simulink model "FPU_sim_out"  (Simulink 7.6)
settings: Solver=FixedStepDiscrete  StartTime=0.0  StopTime=200  FixedStep=1  RelTol=1e-3
libraries: simulink x24
settings Model: Creator=jordan  LastModifiedBy=jordan
settings OptimizationCC: BlockReduction=off  ConditionallyExecuteInputs=off

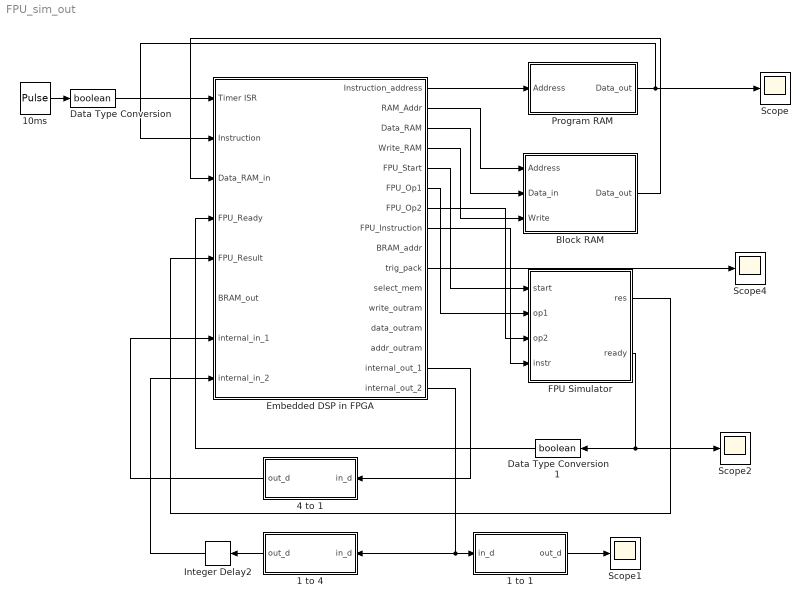
== system FPU_sim_out ==
  1 to 1 : Stateflow chart  TreatAsAtomicUnit=on
  1 to 4 : Stateflow chart  TreatAsAtomicUnit=on
  10ms : DiscretePulseGenerator  Period=50
  4 to 1 : Stateflow chart  TreatAsAtomicUnit=on
  Block RAM : Subsystem
  Data Type Conversion : DataTypeConversion  OutDataTypeStr=boolean
  Data Type Conversion1 : DataTypeConversion  OutDataTypeStr=boolean
  Embedded DSP in FPGA : Subsystem
  FPU Simulator : Stateflow chart  TreatAsAtomicUnit=on
  Integer Delay2 : simulink/Discrete/Integer Delay  NumDelays=1  vinit=0.0  samptime=-1
  Program RAM : Subsystem
  Scope{,1..2,4} (4 alike) : Scope
      Scope settings: MaxDataPoints=50000
      Scope1 settings: SaveName=ScopeData5  MaxDataPoints=50000
      Scope2 settings: SaveName=ScopeData4  MaxDataPoints=50000
      Scope4 settings: SaveName=ScopeData13  MaxDataPoints=50000
  wires:
  10ms/1 -> Data Type Conversion/1
  Data Type Conversion/1 -> Embedded DSP in FPGA/1(Timer ISR)
  Embedded DSP in FPGA/1(Instruction_address) -> Program RAM/1(Address)
  Program RAM/1(Data_out) -> Embedded DSP in FPGA/2(Instruction), Scope/1
  Embedded DSP in FPGA/2(RAM_Addr) -> Block RAM/1(Address)
  Embedded DSP in FPGA/3(Data_RAM) -> Block RAM/2(Data_in)
  Embedded DSP in FPGA/4(Write_RAM) -> Block RAM/3(Write)
  Block RAM/1(Data_out) -> Embedded DSP in FPGA/3(Data_RAM_in)
  Embedded DSP in FPGA/5(FPU_Start) -> FPU Simulator/1(start)
  Embedded DSP in FPGA/6(FPU_Op1) -> FPU Simulator/2(op1)
  Embedded DSP in FPGA/7(FPU_Op2) -> FPU Simulator/3(op2)
  Embedded DSP in FPGA/8(FPU_Instruction) -> FPU Simulator/4(instr)
  FPU Simulator/2(ready) -> Scope2/1, Data Type Conversion1/1
  FPU Simulator/1(res) -> Embedded DSP in FPGA/5(FPU_Result)
  Data Type Conversion1/1 -> Embedded DSP in FPGA/4(FPU_Ready)
  Embedded DSP in FPGA/15(internal_out_1) -> 4 to 1/1(in_d)
  4 to 1/1(out_d) -> Embedded DSP in FPGA/7(internal_in_1)
  Embedded DSP in FPGA/16(internal_out_2) -> 1 to 4/1(in_d), 1 to 1/1(in_d)
  1 to 4/1(out_d) -> Integer Delay2/1
  Integer Delay2/1 -> Embedded DSP in FPGA/8(internal_in_2)
  1 to 1/1(out_d) -> Scope1/1
  Embedded DSP in FPGA/10(trig_pack) -> Scope4/1

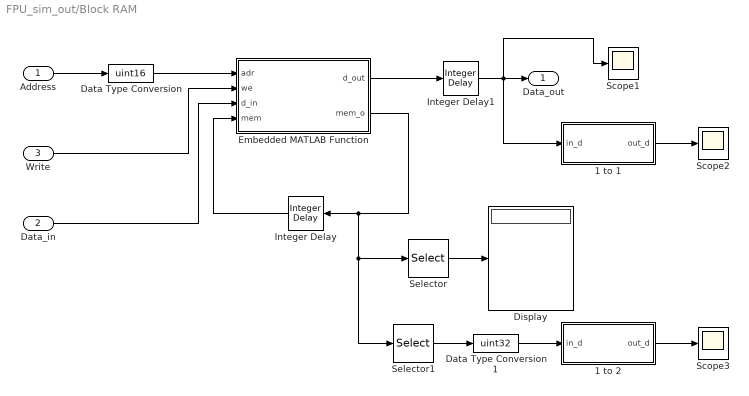
== system FPU_sim_out/Block RAM ==
  Address : Inport  OutDataTypeStr=fixdt(0,12,0)
  Data_in : Inport  Port=2  OutDataTypeStr=uint32
  Write : Inport  Port=3  OutDataTypeStr=boolean
  1 to 1 : Stateflow chart  TreatAsAtomicUnit=on
  1 to 2 : Stateflow chart  TreatAsAtomicUnit=on
  Data Type Conversion : DataTypeConversion  OutDataTypeStr=uint16
  Data Type Conversion1 : DataTypeConversion  OutDataTypeStr=uint32
  Display : Display
  Embedded MATLAB Function : Stateflow chart  TreatAsAtomicUnit=on
  Integer Delay : simulink/Discrete/Integer Delay  NumDelays=1  vinit=zeros(1,100)  samptime=-1
  Integer Delay1 : simulink/Discrete/Integer Delay  NumDelays=1  vinit=0.0  samptime=-1
  Scope1 : Scope
      settings: SaveName=ScopeData23  MaxDataPoints=50000
  Scope2 : Scope
      settings: SaveName=ScopeData14  MaxDataPoints=50000
  Scope3 : Scope
      settings: SaveName=ScopeData31  MaxDataPoints=50000
  Selector : Selector  InputPortWidth=100  IndexOptions=Index vector (dialog)  Indices=1:5  OutputSizes=1
  Selector1 : Selector  InputPortWidth=100  IndexOptions=Index vector (dialog)  Indices=5  OutputSizes=1
  Data_out : Outport  OutDataTypeStr=uint32
  wires:
  Address/1 -> Data Type Conversion/1
  Write/1 -> Embedded MATLAB Function/2(we)
  Data_in/1 -> Embedded MATLAB Function/3(d_in)
  Embedded MATLAB Function/1(d_out) -> Integer Delay1/1
  Integer Delay/1 -> Embedded MATLAB Function/4(mem)
  Embedded MATLAB Function/2(mem_o) -> Integer Delay/1, Selector/1, Selector1/1
  Data Type Conversion/1 -> Embedded MATLAB Function/1(adr)
  Integer Delay1/1 -> Data_out/1, Scope1/1, 1 to 1/1(in_d)
  Selector/1 -> Display/1
  1 to 1/1(out_d) -> Scope2/1
  1 to 2/1(out_d) -> Scope3/1
  Selector1/1 -> Data Type Conversion1/1
  Data Type Conversion1/1 -> 1 to 2/1(in_d)

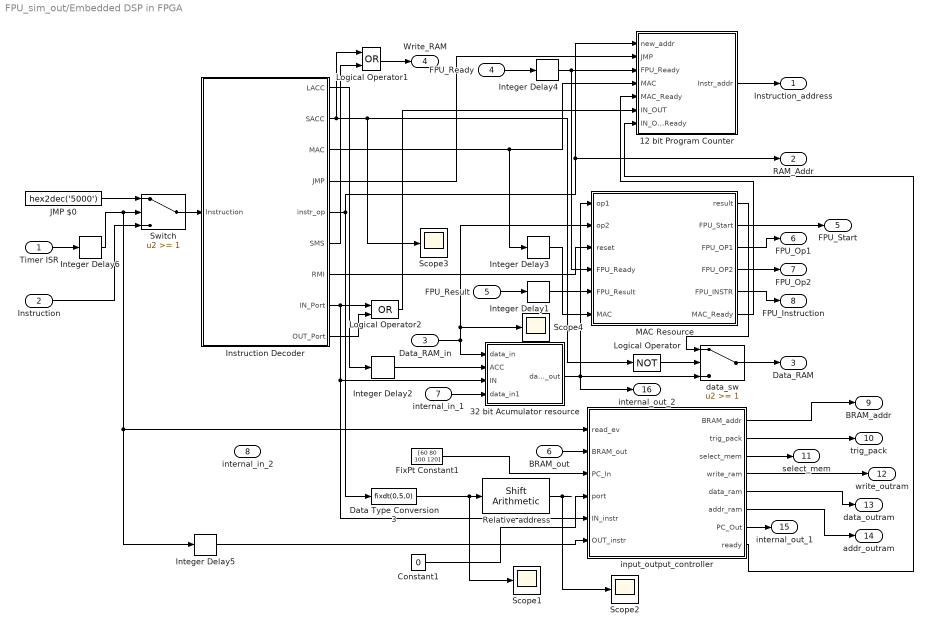
== system FPU_sim_out/Embedded DSP in FPGA ==
  Timer ISR : Inport  OutDataTypeStr=boolean
  Instruction : Inport  Port=2  OutDataTypeStr=uint16
  Data_RAM_in : Inport  Port=3  OutDataTypeStr=uint32
  FPU_Ready : Inport  Port=4  OutDataTypeStr=boolean
  FPU_Result : Inport  Port=5  OutDataTypeStr=uint32
  BRAM_out : Inport  Port=6  OutDataTypeStr=uint8
  internal_in_1 : Inport  Port=7  OutDataTypeStr=uint32
  internal_in_2 : Inport  Port=8
  12 bit Program Counter : Subsystem
  32 bit Acumulator resource : Subsystem
  Constant1 : Constant  Value=0  OutDataTypeStr=fixdt(0,5,0)
  Data Type Conversion3 : DataTypeConversion  OutDataTypeStr=fixdt(0,5,0)
  FixPt Constant1 : Constant  DisableCoverage=on  Value=[60 80 100 120]  OutDataTypeStr=uint8
  Instruction Decoder : Subsystem
  Integer Delay{1..4,6} (5 alike) : simulink/Discrete/Integer Delay  NumDelays=1  vinit=0.0  samptime=-1
  Integer Delay5 : simulink/Discrete/Integer Delay  NumDelays=4  vinit=0.0  samptime=-1
  JMP $0 : Constant  DisableCoverage=on  Value=hex2dec('5000')  OutDataTypeStr=Inherit: Inherit via back propagation
  Logical Operator : Logic  Operator=NOT  AllPortsSameDT=off  OutDataTypeStr=boolean
  Logical Operator1 : Logic  Operator=OR  AllPortsSameDT=off  OutDataTypeStr=boolean
  Logical Operator2 : Logic  Operator=OR  AllPortsSameDT=off  OutDataTypeStr=boolean
  MAC Resource : Stateflow chart  TreatAsAtomicUnit=on
  Relative address : simulink/Logic and Bit Operations/Shift Arithmetic  SystemSampleTime=-1  nBitShiftRight=-2  nBinPtShiftRight=0
  Scope{1..4} (4 alike) : Scope
      Scope1 settings: SaveName=ScopeData18  MaxDataPoints=50000
      Scope2 settings: SaveName=ScopeData17  MaxDataPoints=50000
      Scope3 settings: SaveName=ScopeData25  MaxDataPoints=50000
      Scope4 settings: SaveName=ScopeData24  MaxDataPoints=50000
  Switch : Switch  Threshold=1
  data_sw : Switch  Threshold=1
  input_output_controller : Stateflow chart  TreatAsAtomicUnit=on
  Instruction_address : Outport  OutDataTypeStr=fixdt(0,12,0)
  RAM_Addr : Outport  Port=2  OutDataTypeStr=fixdt(0,12,0)
  Data_RAM : Outport  Port=3  OutDataTypeStr=uint32
  Write_RAM : Outport  Port=4  OutDataTypeStr=boolean
  FPU_Start : Outport  Port=5  OutDataTypeStr=boolean
  FPU_Op1 : Outport  Port=6  OutDataTypeStr=uint32
  FPU_Op2 : Outport  Port=7  OutDataTypeStr=uint32
  FPU_Instruction : Outport  Port=8  OutDataTypeStr=fixdt(0,3,0)
  BRAM_addr : Outport  Port=9
  trig_pack : Outport  Port=10
  select_mem : Outport  Port=11
  write_outram : Outport  Port=12
  data_outram : Outport  Port=13
  addr_outram : Outport  Port=14
  internal_out_1 : Outport  Port=15
  internal_out_2 : Outport  Port=16  OutDataTypeStr=uint32
  wires:
  MAC Resource/1(result) -> data_sw/1
  32 bit Acumulator resource/1(data_out) -> MAC Resource/1(op1), data_sw/3, internal_out_2/1
  Data_RAM_in/1 -> 32 bit Acumulator resource/1(data_in), MAC Resource/2(op2), Scope4/1
  Instruction Decoder/5(instr_op) -> 12 bit Program Counter/1(new_addr), RAM_Addr/1, Data Type Conversion3/1
  Instruction Decoder/1(LACC) -> Integer Delay2/1
  Integer Delay2/1 -> 32 bit Acumulator resource/2(ACC)
  Instruction Decoder/2(SACC) -> Logical Operator1/1, Logical Operator/1, Scope3/1
  Logical Operator/1 -> data_sw/2
  Instruction Decoder/4(JMP) -> 12 bit Program Counter/2(JMP)
  Instruction Decoder/3(MAC) -> Integer Delay3/1, 12 bit Program Counter/4(MAC)
  Integer Delay3/1 -> MAC Resource/6(MAC)
  Instruction Decoder/7(RMI) -> MAC Resource/3(reset)
  Instruction Decoder/6(SMS) -> Logical Operator1/2
  Instruction Decoder/8(IN_Port) -> input_output_controller/5(IN_instr), 32 bit Acumulator resource/3(IN), Logical Operator2/1
  Data Type Conversion3/1 -> Relative address/1, Scope1/1
  Switch/1 -> Instruction Decoder/1(Instruction)
  JMP $0/1 -> Switch/1
  12 bit Program Counter/1(Instr_addr) -> Instruction_address/1
  Timer ISR/1 -> Integer Delay6/1
  Instruction/1 -> Switch/3
  data_sw/1 -> Data_RAM/1
  Logical Operator1/1 -> Write_RAM/1
  FPU_Ready/1 -> Integer Delay4/1
  FPU_Result/1 -> Integer Delay1/1
  MAC Resource/3(FPU_OP1) -> FPU_Op1/1
  MAC Resource/4(FPU_OP2) -> FPU_Op2/1
  MAC Resource/5(FPU_INSTR) -> FPU_Instruction/1
  MAC Resource/2(FPU_Start) -> FPU_Start/1
  Integer Delay4/1 -> 12 bit Program Counter/3(FPU_Ready), MAC Resource/4(FPU_Ready)
  Instruction Decoder/9(OUT_Port) -> Logical Operator2/2
  BRAM_out/1 -> input_output_controller/2(BRAM_out)
  input_output_controller/6(addr_ram) -> addr_outram/1
  input_output_controller/4(write_ram) -> write_outram/1
  input_output_controller/5(data_ram) -> data_outram/1
  input_output_controller/1(BRAM_addr) -> BRAM_addr/1
  input_output_controller/2(trig_pack) -> trig_pack/1
  input_output_controller/3(select_mem) -> select_mem/1
  Relative address/1 -> Scope2/1
  input_output_controller/8(ready) -> 12 bit Program Counter/7(IN_OUT_Ready)
  MAC Resource/6(MAC_Ready) -> 12 bit Program Counter/5(MAC_Ready)
  Logical Operator2/1 -> 12 bit Program Counter/6(IN_OUT)
  input_output_controller/7(PC_Out) -> internal_out_1/1
  internal_in_1/1 -> 32 bit Acumulator resource/4(data_in1)
  Integer Delay1/1 -> MAC Resource/5(FPU_Result)
  FixPt Constant1/1 -> input_output_controller/3(PC_In)
  Constant1/1 -> input_output_controller/4(port)
  Integer Delay6/1 -> Switch/2, input_output_controller/1(read_ev), Integer Delay5/1
  Integer Delay5/1 -> input_output_controller/6(OUT_instr)

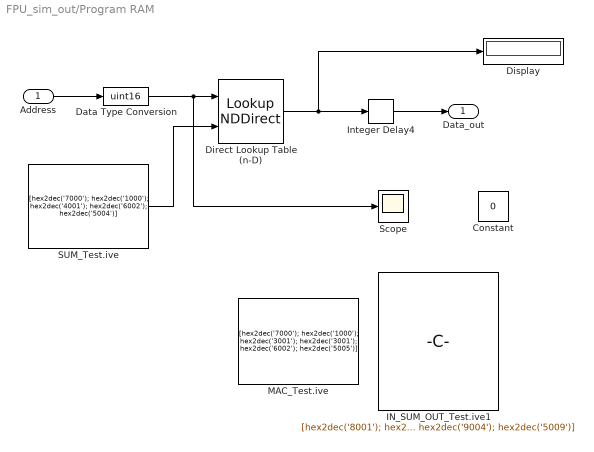
== system FPU_sim_out/Program RAM ==
  Address : Inport
  Constant : Constant  Value=0
  Data Type Conversion : DataTypeConversion  OutDataTypeStr=uint16
  Direct Lookup Table (n-D) : LookupNDDirect  NumberOfTableDimensions=1  TableIsInput=on  Table=[hex2dec('1000') hex2dec('4001') hex2dec('2002') hex2dec('5003')]  SampleTime=1  TableDataTypeStr=uint16
  Display : Display
      settings: Format=hex (Stored Integer)
  IN_SUM_OUT_Test.ive1 : Constant  Value=[hex2dec('8001'); hex2dec('2000'); hex2dec('8002'); hex2dec('2001'); hex2dec('1000'); hex2dec('4001'); hex2dec('6002'); hex2dec('1002'); hex2dec('9004'); hex2dec('5009')]  VectorParams1D=off  OutDataTypeStr=uint16
  Integer Delay4 : simulink/Discrete/Integer Delay  NumDelays=1  vinit=0.0  samptime=-1
  MAC_Test.ive : Constant  Value=[hex2dec('7000'); hex2dec('1000'); hex2dec('3001'); hex2dec('3001'); hex2dec('6002'); hex2dec('5005')]  VectorParams1D=off  OutDataTypeStr=uint16
  SUM_Test.ive : Constant  Value=[hex2dec('7000'); hex2dec('1000'); hex2dec('4001'); hex2dec('6002'); hex2dec('5004')]  VectorParams1D=off  OutDataTypeStr=uint16
  Scope : Scope
      settings: MaxDataPoints=50000
  Data_out : Outport
  wires:
  Address/1 -> Data Type Conversion/1
  Direct Lookup Table (n-D)/1 -> Display/1, Integer Delay4/1
  SUM_Test.ive/1 -> Direct Lookup Table (n-D)/2
  Integer Delay4/1 -> Data_out/1
  Data Type Conversion/1 -> Direct Lookup Table (n-D)/1, Scope/1

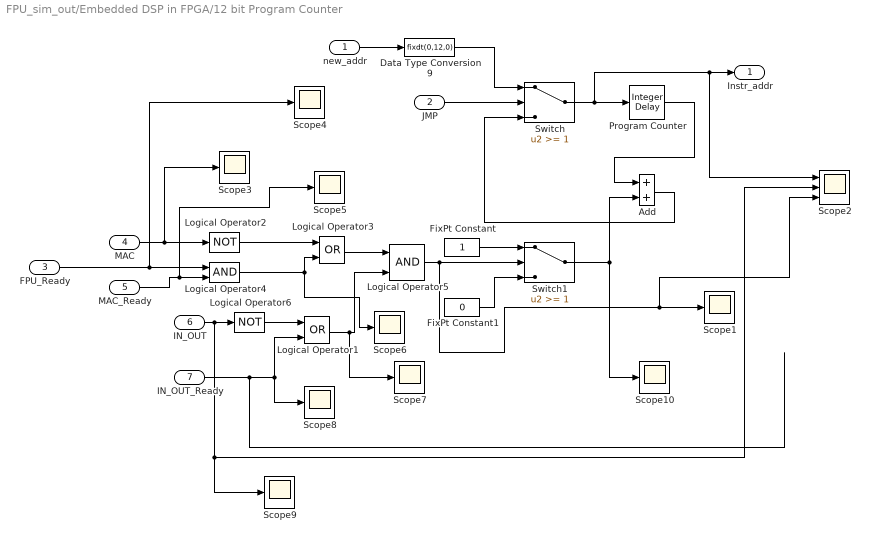
== system FPU_sim_out/Embedded DSP in FPGA/12 bit Program Counter ==
  new_addr : Inport
  JMP : Inport  Port=2
  FPU_Ready : Inport  Port=3  OutDataTypeStr=boolean
  MAC : Inport  Port=4  OutDataTypeStr=boolean
  MAC_Ready : Inport  Port=5  OutDataTypeStr=boolean
  IN_OUT : Inport  Port=6  OutDataTypeStr=boolean
  IN_OUT_Ready : Inport  Port=7  OutDataTypeStr=boolean
  Add : Sum  AccumDataTypeStr=fixdt(0,12,0)  OutDataTypeStr=fixdt(0,12,0)
  Data Type Conversion9 : DataTypeConversion  OutDataTypeStr=fixdt(0,12,0)
  FixPt Constant : Constant  DisableCoverage=on  OutDataTypeStr=fixdt(0,12,0)
  FixPt Constant1 : Constant  DisableCoverage=on  Value=0  OutDataTypeStr=fixdt(0,12,0)
  Logical Operator1 : Logic  Operator=OR  AllPortsSameDT=off  OutDataTypeStr=boolean
  Logical Operator2 : Logic  Operator=NOT  AllPortsSameDT=off  OutDataTypeStr=boolean
  Logical Operator3 : Logic  Operator=OR  AllPortsSameDT=off  OutDataTypeStr=boolean
  Logical Operator4 : Logic  AllPortsSameDT=off  OutDataTypeStr=boolean
  Logical Operator5 : Logic  AllPortsSameDT=off  OutDataTypeStr=boolean
  Logical Operator6 : Logic  Operator=NOT  AllPortsSameDT=off  OutDataTypeStr=boolean
  Program Counter : simulink/Discrete/Integer Delay  NumDelays=1  vinit=0.0  samptime=-1
  Scope{1,3..10} (9 alike) : Scope
      Scope1 settings: SaveName=ScopeData2
      Scope10 settings: SaveName=ScopeData16
      Scope3 settings: SaveName=ScopeData6
      Scope4 settings: SaveName=ScopeData7
      Scope5 settings: SaveName=ScopeData8
      Scope6 settings: SaveName=ScopeData9
      Scope7 settings: SaveName=ScopeData10
      Scope8 settings: SaveName=ScopeData11
      Scope9 settings: SaveName=ScopeData12
  Scope2 : Scope  NumInputPorts=3
      settings: YMin=-5~-5~-5  YMax=5~5~5  SaveName=ScopeData3
  Switch : Switch  Threshold=1
  Switch1 : Switch  Threshold=1
  Instr_addr : Outport  InitialOutput=0
  wires:
  JMP/1 -> Switch/2
  new_addr/1 -> Data Type Conversion9/1
  Program Counter/1 -> Add/1
  Switch/1 -> Program Counter/1, Instr_addr/1, Scope2/1
  FixPt Constant/1 -> Switch1/1
  Add/1 -> Switch/3
  Data Type Conversion9/1 -> Switch/1
  Switch1/1 -> Add/2, Scope10/1
  FixPt Constant1/1 -> Switch1/3
  Logical Operator5/1 -> Switch1/2, Scope1/1, Scope2/3
  FPU_Ready/1 -> Logical Operator4/1, Scope4/1
  Logical Operator4/1 -> Logical Operator3/2, Scope6/1
  Logical Operator3/1 -> Logical Operator5/1
  Logical Operator2/1 -> Logical Operator3/1
  MAC/1 -> Logical Operator2/1, Scope3/1
  MAC_Ready/1 -> Logical Operator4/2, Scope5/1
  Logical Operator1/1 -> Logical Operator5/2, Scope7/1
  Logical Operator6/1 -> Logical Operator1/1
  IN_OUT/1 -> Logical Operator6/1, Scope9/1, Scope2/2
  IN_OUT_Ready/1 -> Logical Operator1/2, Scope8/1

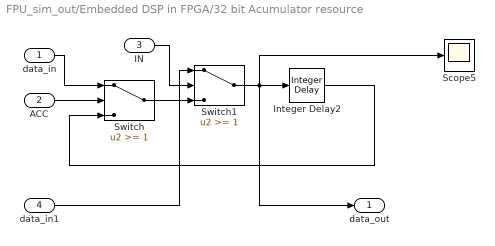
== system FPU_sim_out/Embedded DSP in FPGA/32 bit Acumulator resource ==
  data_in : Inport
  ACC : Inport  Port=2
  IN : Inport  Port=3
  data_in1 : Inport  Port=4
  Integer Delay2 : simulink/Discrete/Integer Delay  NumDelays=1  vinit=0.0  samptime=-1
  Scope5 : Scope
      settings: SaveName=ScopeData21  MaxDataPoints=50000
  Switch : Switch  Threshold=1
  Switch1 : Switch  Threshold=1
  data_out : Outport  OutDataTypeStr=uint32
  wires:
  Switch/1 -> Switch1/3
  Integer Delay2/1 -> Switch/3
  data_in/1 -> Switch/1
  ACC/1 -> Switch/2
  Switch1/1 -> Integer Delay2/1, data_out/1, Scope5/1
  IN/1 -> Switch1/2
  data_in1/1 -> Switch1/1

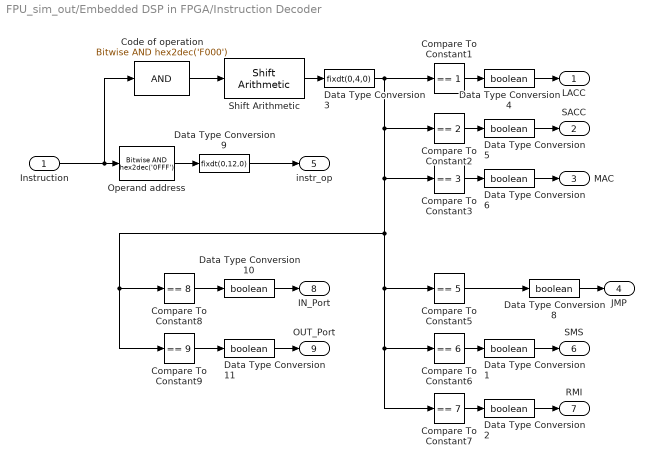
== system FPU_sim_out/Embedded DSP in FPGA/Instruction Decoder ==
  Instruction : Inport  OutDataTypeStr=uint16
  Code of operation : simulink/Logic and Bit Operations/Bitwise Operator  logicop=AND  UseBitMask=on  BitMask=hex2dec('F000')  BitMaskRealWorld=Stored Integer
  Compare To Constant1 : simulink/Logic and Bit Operations/Compare To Constant  SystemSampleTime=-1  relop===  const=1  LogicOutDataTypeMode=boolean
  Compare To Constant2 : simulink/Logic and Bit Operations/Compare To Constant  SystemSampleTime=-1  relop===  const=2  LogicOutDataTypeMode=boolean
  Compare To Constant3 : simulink/Logic and Bit Operations/Compare To Constant  SystemSampleTime=-1  relop===  const=3  LogicOutDataTypeMode=boolean
  Compare To Constant5 : simulink/Logic and Bit Operations/Compare To Constant  SystemSampleTime=-1  relop===  const=5  LogicOutDataTypeMode=boolean
  Compare To Constant6 : simulink/Logic and Bit Operations/Compare To Constant  SystemSampleTime=-1  relop===  const=6  LogicOutDataTypeMode=boolean
  Compare To Constant7 : simulink/Logic and Bit Operations/Compare To Constant  SystemSampleTime=-1  relop===  const=7  LogicOutDataTypeMode=boolean
  Compare To Constant8 : simulink/Logic and Bit Operations/Compare To Constant  SystemSampleTime=-1  relop===  const=8  LogicOutDataTypeMode=boolean
  Compare To Constant9 : simulink/Logic and Bit Operations/Compare To Constant  SystemSampleTime=-1  relop===  const=9  LogicOutDataTypeMode=boolean
  Data Type Conversion{1..2,4..6,8,10..11} (8 alike) : DataTypeConversion  OutDataTypeStr=boolean
  Data Type Conversion3 : DataTypeConversion  OutDataTypeStr=fixdt(0,4,0)
  Data Type Conversion9 : DataTypeConversion  OutDataTypeStr=fixdt(0,12,0)
  Operand address : simulink/Logic and Bit Operations/Bitwise Operator  logicop=AND  UseBitMask=on  BitMask=hex2dec('0FFF')  BitMaskRealWorld=Stored Integer
  Shift Arithmetic : simulink/Logic and Bit Operations/Shift Arithmetic  SystemSampleTime=-1  nBitShiftRight=12  nBinPtShiftRight=0
  LACC : Outport
  SACC : Outport  Port=2
  MAC : Outport  Port=3
  JMP : Outport  Port=4
  instr_op : Outport  Port=5
  SMS : Outport  Port=6
  RMI : Outport  Port=7
  IN_Port : Outport  Port=8
  OUT_Port : Outport  Port=9
  wires:
  Instruction/1 -> Operand address/1, Code of operation/1
  Code of operation/1 -> Shift Arithmetic/1
  Shift Arithmetic/1 -> Data Type Conversion3/1
  Data Type Conversion3/1 -> Compare To Constant6/1, Compare To Constant7/1, Compare To Constant5/1, Compare To Constant8/1, Compare To Constant9/1, Compare To Constant3/1, Compare To Constant2/1, Compare To Constant1/1
  Compare To Constant1/1 -> Data Type Conversion4/1
  Compare To Constant2/1 -> Data Type Conversion5/1
  Compare To Constant3/1 -> Data Type Conversion6/1
  Compare To Constant5/1 -> Data Type Conversion8/1
  Operand address/1 -> Data Type Conversion9/1
  Data Type Conversion4/1 -> LACC/1
  Data Type Conversion5/1 -> SACC/1
  Data Type Conversion9/1 -> instr_op/1
  Data Type Conversion6/1 -> MAC/1
  Data Type Conversion8/1 -> JMP/1
  Compare To Constant6/1 -> Data Type Conversion1/1
  Data Type Conversion1/1 -> SMS/1
  Compare To Constant7/1 -> Data Type Conversion2/1
  Data Type Conversion2/1 -> RMI/1
  Compare To Constant8/1 -> Data Type Conversion10/1
  Data Type Conversion10/1 -> IN_Port/1
  Compare To Constant9/1 -> Data Type Conversion11/1
  Data Type Conversion11/1 -> OUT_Port/1

== matlab function 4 to 1 ==
  data: out_d output uint32; in_d input uint8 size=4
function out_d  = fcn(in_d)
%#eml
out_d=uint32(bitor(bitor(bitor(in_d(1),bitshift(in_d(2),8)),bitshift(in_d(3),16)),bitshift(in_d(4),24)));

== matlab function Block RAM/Embedded MATLAB Function ==
  data: adr input double; d_out output uint32; we input double; d_in input double; mem input double size=100; mem_o output double size=100
function [d_out,mem_o] = fcn(adr,we,d_in,mem)
%#eml

if (adr<100)
        d_out=uint32(mem(adr+1));
    if (we==1)
        mem(adr+1)=d_in;
    end
else
    d_out=uint32(0);
end
mem_o=mem;

== stateflow chart Embedded DSP in FPGA/MAC Resource ==
  settings: executeAtInitialization=1
  state Multipy
  state Accumulate
  state Wait
  state Wait1
  state Wait2
  (default) -> Wait
  (junction 26) -> Multipy [order 2] : [MAC]{
      | FPU_OP1=op1;
      | FPU_OP2=op2;
      | FPU_INSTR=2;
      | FPU_Start=1;}
  Multipy -> Wait1 : [FPU_Ready]{
      | FPU_OP1=FPU_Result;
      | FPU_Start=0;}
  Wait1 -> Accumulate : {FPU_OP2=Internal_ACC;
      | FPU_INSTR=0;
      | FPU_Start=1;}
  Accumulate -> Wait2 : [FPU_Ready]{
      | FPU_Start=0;
      | Internal_ACC=FPU_Result;
      | result=Internal_ACC;
      | MAC_Ready=1;}
  Wait -> (junction 26) : {MAC_Ready=0;}
  (junction 26) -> Wait [order 1] : [reset]{
      | Internal_ACC=0;}
  (junction 26) -> Wait [order 3]
  Wait2 -> Wait
  data: op1 input uint32; op2 input uint32; reset input boolean; Internal_ACC local uint32; result output uint32; FPU_Start output boolean; FPU_Ready input boolean; FPU_OP1 output uint32; FPU_OP2 output uint32; FPU_Result input uint32; FPU_INSTR output fixdt(0,3,0); MAC input boolean; MAC_Ready output boolean

== stateflow chart Embedded DSP in FPGA/input_output_controller ==
  settings: executeAtInitialization=1
  state IN_Wait
  state Receive
  state OUT_Wait
  state Wait2
  state Wait3
  state Wait
  state Wait4
  (default) -> Receive
  (junction 59) -> Wait4 [order 1] : [ind==4]{ready=1;}
  Wait2 -> Receive : {trig_pack=0;}
  (junction 60) -> Wait4 [order 1] : [ind==4]{
      | write_ram=0;
      | ready=1;}
  (junction 59) -> IN_Wait [order 2]
  Receive -> Wait3 [order 3] : [read_ev==1]{
      | BRAM_addr=14;}
  IN_Wait -> (junction 59) : {PC_Out[ind]=BRAM_out;
      | ind++;
      | BRAM_addr=BRAM_addr+1;}
  (junction 60) -> OUT_Wait [order 2] : {addr_ram=addr_ram+1;
      | data_ram=PC_In[ind];}
  OUT_Wait -> (junction 60) : {ind++;}
  (junction 61) -> Wait2 : {trig_pack=1;}
  (junction 58) -> (junction 61) [order 2] : {select_mem=2;}/*Data Packet*/
  Wait -> OUT_Wait : {addr_ram=port;
      | write_ram=1;
      | data_ram=PC_In[0];
      | ind=0;}
  Wait3 -> (junction 58)
  Receive -> IN_Wait [order 2] : [IN_instr==1]{
      | BRAM_addr=46+port;
      | ind=0;
      | ready=0;}
  (junction 58) -> (junction 61) [order 1] : [BRAM_out==6]{
      | select_mem=4;}
      | /*ARP Request*/
  Receive -> Wait [order 1] : [OUT_instr==1]{ready=0;}
  Wait4 -> Receive : {ready=0;}
  data: read_ev input boolean; BRAM_out input uint8; BRAM_addr output fixdt(0,11,0) =0; trig_pack output boolean; select_mem output fixdt(0,4,0) =0; ind local fixdt(0,5,0) =0; LastCmd local uint8; packet_out local uint8 size=16; write_ram output boolean =0; data_ram output uint8; addr_ram output fixdt(0,14,0) =0; PC_In input uint8 size=4; PC_Out output uint8 size=4; port input fixdt(0,5,0); IN_instr input boolean; ready output boolean; OUT_instr input boolean

== matlab function FPU Simulator ==
  data: res output uint32; start input boolean; op1 input uint32; op2 input uint32; instr input double; ready output boolean
function [res,ready]  = fcn(start,op1,op2,instr)
%#eml
res=uint32(0);
ready=0;
if (start==1)
    op1s=typecast(op1,'single');
    op2s=typecast(op2,'single');
    if (instr==0)
        res_s=single(op1s+op2s);
        res=typecast(res_s,'uint32');
        ready=1;
    end
    if (instr==2)
        res_s=single(op1s*op2s);
        res=typecast(res_s,'uint32');
        ready=1;
    end
end

== matlab function 1 to 4 ==
  data: out_d output uint8; in_d input uint32
function out_d  = fcn(in_d)
%#eml
out_d=typecast(in_d,'uint8');

== matlab function 1 to 1 ==
  data: out_d output single; in_d input uint32 size=1
function out_d  = fcn(in_d)
%#eml
out_d=typecast(in_d,'single');

== matlab function Block RAM/1 to 1 ==
  data: out_d output single; in_d input uint32 size=1
function out_d  = fcn(in_d)
%#eml
out_d=typecast(in_d,'single');

== matlab function Block RAM/1 to 2 ==
  data: out_d output single; in_d input uint32 size=1
function out_d  = fcn(in_d)
%#eml
out_d=typecast(in_d,'single');
